simulink model "Total_B2B_latest"  (R2018a)
settings: Solver=ode8  StartTime=0.0  StopTime=10  FixedStep=20e-6  RelTol=1e-3
values from neighbouring files (symbols this model uses):
  A = R^2*pi    (= 24996.5217713)    [Total_init.m]    (also in Total_init_trafo.m)
  C1 = 0.0117    [Total_init.m]    (also in Total_init_trafo.m)
  C2 = 5500    [Total_init.m]    (also in Total_init_trafo.m)
  C3 = 10    [Total_init.m]    (also in Total_init_trafo.m)
  C4 = 0    [Total_init.m]    (also in Total_init_trafo.m)
  C5 = 160    [Total_init.m]    (also in Total_init_trafo.m)
  C6 = 23.38    [Total_init.m]    (also in Total_init_trafo.m)
  C_dc = 1e-2    (= 0.01)    [Total_init.m]    (also in Total_init_trafo.m)
  Cx = 0    [Total_init.m]    (also in Total_init_trafo.m)
  fg = 50    [Total_init.m]    (also in Total_init_trafo.m)
  Ir = 2*Pr/(3*Er*cosphi)    (= 2057.61316872)    [Total_init.m]    (also in Total_init_trafo.m)
  J = 12.8e6    (= 12800000)    [Total_init.m]    (also in Total_init_trafo.m)
  Jr = 3*m*r^2    (= 105248711.1)    [Total_init.m]    (also in Total_init_trafo.m)
  KI_d = KP_d*Rs/Ld    (= 1454)    [Total_init.m]    (also in Total_init_trafo.m)
  KP_d = 50    [Total_init.m]    (also in Total_init_trafo.m)
  KP_g = 5    [Total_init.m]    (also in Total_init_trafo.m)
  KP_gv = 5    [Total_init.m]    (also in Total_init_trafo.m)
  lambda_m = Er/(om_r*p)    (= 21.4859173174)    [Total_init.m]    (also in Total_init_trafo.m)
  lambda_opt = 9.35    [Total_init.m]    (also in Total_init_trafo.m)
  Ld = 0.005    [Total_init.m]    (also in Total_init_trafo.m)
  Lg = 1e-3    (= 0.001)    [Total_init.m]    (also in Total_init_trafo.m)
  Linvmat = Lmat^(-1)    [Total_init.m]    (also in Total_init_trafo.m)
  Lq = 0.005    [Total_init.m]    (also in Total_init_trafo.m)
  om0 = om_r    (= 1.0471975512)    [Total_init.m]    (also in Total_init_trafo.m)
  om_g = 100*pi    (= 314.159265359)    [Total_init.m]    (also in Total_init_trafo.m)
  om_r = 10/60*2*pi    (= 1.0471975512)    [Total_init.m]    (also in Total_init_trafo.m)
  p = 160    [Total_init.m]    (also in Total_init_trafo.m)
  Pr = 10e6    (= 10000000)    [Total_init.m]    (also in Total_init_trafo.m)
  psi0 = Lmat*I0'+psif    [Total_init.m]    (also in Total_init_trafo.m)
  psif = [lambda_m; 0]    [Total_init.m]    (also in Total_init_trafo.m)
  R = 89.2    [Total_init.m]    (also in Total_init_trafo.m)
  R_cs = 1e9    (= 1000000000)    [Total_init.m]    (also in Total_init_trafo.m)
  R_dc = 1e-3    (= 0.001)    [Total_init.m]    (also in Total_init_trafo.m)
  Rg = 1e-6    (= 1e-06)    [Total_init.m]    (also in Total_init_trafo.m)
  rho = 1.225    [Total_init.m]    (also in Total_init_trafo.m)
  Rmat = [Rs 0;         0 Rs]    [Total_init.m]    (also in Total_init_trafo.m)
  Rs = 0.1454    [Total_init.m]    (also in Total_init_trafo.m)
  ts = 0.0001    [Total_init.m]    (also in Total_init_trafo.m)
  Vac = 4000    [Total_init.m]    (also in Total_init_trafo.m)
  Vdc = Vac*sqrt(3)    [Total_init.m]    (also in Total_init_trafo.m)
  Vgsc = Vac    (= 4000)    [Total_init.m]    (also in Total_init_trafo.m)
libraries: powerlib x18, simulink x9
(part 2 of 2)

== system Total_B2B_latest/B2B+grid/MSC/MSC_Controller/Iq_Control ==
  real : Inport
  ref : Inport  Port=2
  Integrator : Integrator  LimitOutput=on  UpperSaturationLimit=Vac  LowerSaturationLimit=-Vac
  K_I : Gain  Gain=10*Rs/Lq
  K_P : Gain  Gain=10
  Saturation : Saturate  UpperLimit=Vac  LowerLimit=-Vac
  Sum : Sum  Inputs=|-+
  Sum1 : Sum  Inputs=|++
  TuneScope_Iq : Scope  NumInputPorts=3
  out : Outport
  wires:
  real/1 -> TuneScope_Iq/1, Sum/1
  K_I/1 -> Integrator/1
  Sum/1 -> K_P/1, K_I/1
  Integrator/1 -> Sum1/1
  Sum1/1 -> Saturation/1
  K_P/1 -> Sum1/2
  Saturation/1 -> TuneScope_Iq/3, out/1
  ref/1 -> TuneScope_Iq/2, Sum/2

== system Total_B2B_latest/B2B+grid/MSC/MSC_Controller/Modulator ==
  v_albe : Inport
  Add : Sum
  Add1 : Sum  Inputs=-+
  Add2 : Sum  Inputs=+-
  Carrier Wave : simulink/Sources/Repeating Sequence  rep_seq_t=[0 0.5/Fs 1/Fs]  rep_seq_y=[-1 1 -1]
  Compare To Zero : simulink/Logic and Bit Operations/Compare To Zero  relop=>=  OutDataTypeStr=boolean
  Constant : Constant  Value=Vdc/2
  Data Type Conversion : DataTypeConversion
  Gain2 : Gain  Gain=0.5
  Gate assignment : Subsystem
  Product : Product
  albe2abc : Subsystem
  max : MinMax  Function=max
  min : MinMax
  Out1 : Outport
  wires:
  Gate assignment/1(G) -> Out1/1
  min/1 -> Add/2
  max/1 -> Add/1
  Add/1 -> Gain2/1
  Gain2/1 -> Add1/1
  Add2/1 -> Compare To Zero/1
  Constant/1 -> Product/2
  Carrier Wave/1 -> Product/1
  albe2abc/1(abc) -> Add1/2, min/1, max/1
  Product/1 -> Add2/2
  v_albe/1 -> albe2abc/1(a+bj)
  Compare To Zero/1 -> Data Type Conversion/1
  Data Type Conversion/1 -> Gate assignment/1(E)
  Add1/1 -> Add2/1

== system Total_B2B_latest/B2B+grid/MSC/MSC_Controller/Speed_Control ==
  ref : Inport
  real : Inport  Port=2
  Integrator : Integrator  LimitOutput=on  UpperSaturationLimit=Ir  LowerSaturationLimit=-Ir
  K_I : Gain  Gain=1e4
  K_P : Gain  Gain=2e4
  Saturation : Saturate  UpperLimit=Ir  LowerLimit=-Ir
  Sum : Sum  Inputs=|-+
  Sum1 : Sum  Inputs=|++
  TuneScope_w : Scope  NumInputPorts=3
  out : Outport
  wires:
  ref/1 -> Sum/2, TuneScope_w/1
  real/1 -> TuneScope_w/2, Sum/1
  K_I/1 -> Integrator/1
  Sum/1 -> K_P/1, K_I/1
  Integrator/1 -> Sum1/1
  Sum1/1 -> Saturation/1
  K_P/1 -> Sum1/2
  Saturation/1 -> TuneScope_w/3, out/1

== system Total_B2B_latest/B2B+grid/GSC/GSC_Modulator1/Modulator/Gate assignment ==
  E : Inport
  Constant : Constant
  Demux : Demux  Outputs=3
  Demux1 : Demux  Outputs=3
  Mux : Mux  Inputs=6
  Sum1 : Sum  Inputs=-+|  SaturateOnIntegerOverflow=on  InputSameDT=on  OutDataTypeStr=Inherit: Same as first input
  G : Outport
  wires:
  Demux/3 -> Mux/5  "C(high)"
  Demux1/3 -> Mux/6  "C(low)"
  Mux/1 -> G/1
  Sum1/1 -> Demux1/1
  E/1 -> Sum1/1, Demux/1
  Constant/1 -> Sum1/2
  Demux/1 -> Mux/1  "A(high)"
  Demux/2 -> Mux/3  "B(high)"
  Demux1/2 -> Mux/4  "B(low)"
  Demux1/1 -> Mux/2  "A(low)"

== system Total_B2B_latest/B2B+grid/GSC/GSC_Modulator1/Modulator/albe2abc ==
  a+bj : Inport
  Gain : Gain  Gain=[1, 0; -0.5, sqrt(3)/2; -0.5, -sqrt(3)/2 ]  Multiplication=Matrix(K*u) (u vector)
  abc : Outport
  wires:
  Gain/1 -> abc/1
  a+bj/1 -> Gain/1

== system Total_B2B_latest/B2B+grid/GSC/GSC_Modulator1/abc->dq/C_rot ==
  in_1 : Inport
  in_3 : Inport  Port=2
  Demux : Demux  Outputs=2
  Product{,1..3} (4 alike) : Product  SaturateOnIntegerOverflow=on  RndMeth=Zero  InputSameDT=on  OutDataTypeStr=Inherit: Same as first input
  Sum : Sum  Inputs=+-  SaturateOnIntegerOverflow=on  InputSameDT=on  OutDataTypeStr=Inherit: Same as first input
  Sum1 : Sum  SaturateOnIntegerOverflow=on  InputSameDT=on  OutDataTypeStr=Inherit: Same as first input
  cos : Fcn  Expr=cos(u(1))
  sin : Fcn  Expr=sin(u(1))
  out_1 : Outport
  out_2 : Outport  Port=2
  wires:
  Demux/2 -> Product/1, Product2/1
  Demux/1 -> Product3/1, Product1/1
  Sum1/1 -> out_2/1
  Sum/1 -> out_1/1
  cos/1 -> Product/2, Product1/2
  sin/1 -> Product3/2, Product2/2
  in_3/1 -> sin/1, cos/1
  Product/1 -> Sum1/2
  Product1/1 -> Sum/1
  Product3/1 -> Sum1/1
  Product2/1 -> Sum/2
  in_1/1 -> Demux/1

== system Total_B2B_latest/B2B+grid/GSC/GSC_Modulator1/abc->dq/abc-ab ==
  abc : Inport
  3 naar 2 : Subsystem
  Demux : Demux  Outputs=3
  Mux : Mux  Inputs=2
  ab : Outport
  wires:
  abc/1 -> Demux/1
  Demux/1 -> 3 naar 2/1(in_1)
  Demux/2 -> 3 naar 2/2(in_2)
  Demux/3 -> 3 naar 2/3(in_3)
  3 naar 2/1(out_1) -> Mux/1
  3 naar 2/2(out_2) -> Mux/2
  Mux/1 -> ab/1

== system Total_B2B_latest/B2B+grid/GSC/GSC_Modulator1/abc->dq1/C_rot ==
  in_1 : Inport
  in_3 : Inport  Port=2
  Demux : Demux  Outputs=2
  Product{,1..3} (4 alike) : Product  SaturateOnIntegerOverflow=on  RndMeth=Zero  InputSameDT=on  OutDataTypeStr=Inherit: Same as first input
  Sum : Sum  Inputs=+-  SaturateOnIntegerOverflow=on  InputSameDT=on  OutDataTypeStr=Inherit: Same as first input
  Sum1 : Sum  SaturateOnIntegerOverflow=on  InputSameDT=on  OutDataTypeStr=Inherit: Same as first input
  cos : Fcn  Expr=cos(u(1))
  sin : Fcn  Expr=sin(u(1))
  out_1 : Outport
  out_2 : Outport  Port=2
  wires:
  Demux/2 -> Product/1, Product2/1
  Demux/1 -> Product3/1, Product1/1
  Sum1/1 -> out_2/1
  Sum/1 -> out_1/1
  cos/1 -> Product/2, Product1/2
  sin/1 -> Product3/2, Product2/2
  in_3/1 -> sin/1, cos/1
  Product/1 -> Sum1/2
  Product1/1 -> Sum/1
  Product3/1 -> Sum1/1
  Product2/1 -> Sum/2
  in_1/1 -> Demux/1

== system Total_B2B_latest/B2B+grid/GSC/GSC_Modulator1/abc->dq1/abc-ab ==
  abc : Inport
  3 naar 2 : Subsystem
  Demux : Demux  Outputs=3
  Mux : Mux  Inputs=2
  ab : Outport
  wires:
  abc/1 -> Demux/1
  Demux/1 -> 3 naar 2/1(in_1)
  Demux/2 -> 3 naar 2/2(in_2)
  Demux/3 -> 3 naar 2/3(in_3)
  3 naar 2/1(out_1) -> Mux/1
  3 naar 2/2(out_2) -> Mux/2
  Mux/1 -> ab/1

== system Total_B2B_latest/B2B+grid/GSC/GSC_Modulator1/dq->ab/C_rot ==
  in_1 : Inport
  in_3 : Inport  Port=2
  Demux : Demux  Outputs=2
  Product{,1..3} (4 alike) : Product  SaturateOnIntegerOverflow=on  RndMeth=Zero  InputSameDT=on  OutDataTypeStr=Inherit: Same as first input
  Sum : Sum  Inputs=+-  SaturateOnIntegerOverflow=on  InputSameDT=on  OutDataTypeStr=Inherit: Same as first input
  Sum1 : Sum  SaturateOnIntegerOverflow=on  InputSameDT=on  OutDataTypeStr=Inherit: Same as first input
  cos : Fcn  Expr=cos(u(1))
  sin : Fcn  Expr=sin(u(1))
  out_1 : Outport
  out_2 : Outport  Port=2
  wires:
  Demux/2 -> Product/1, Product2/1
  Demux/1 -> Product3/1, Product1/1
  Sum1/1 -> out_2/1
  Sum/1 -> out_1/1
  cos/1 -> Product/2, Product1/2
  sin/1 -> Product3/2, Product2/2
  in_3/1 -> sin/1, cos/1
  Product/1 -> Sum1/2
  Product1/1 -> Sum/1
  Product3/1 -> Sum1/1
  Product2/1 -> Sum/2
  in_1/1 -> Demux/1

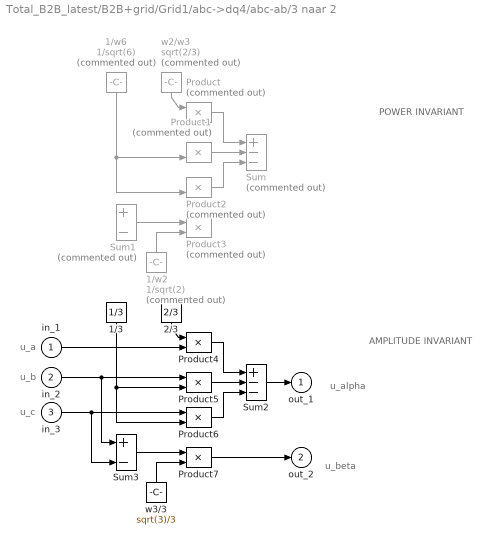
== system Total_B2B_latest/B2B+grid/Grid1/abc->dq4/abc-ab/3 naar 2 ==
  note: POWER INVARIANT
  note: AMPLITUDE INVARIANT
  note: u_beta
  note: u_alpha
  note: u_a
  note: u_c
  note: u_b
  in_1 : Inport
  in_2 : Inport  Port=2
  in_3 : Inport  Port=3
  1/3 : Constant  Value=1/3
  1/w2 : Constant  Commented=on  Value=1/sqrt(2)
  1/w6 : Constant  Commented=on  Value=1/sqrt(6)
  2/3 : Constant  Value=2/3
  Product{,1..3} (4 alike) : Product  Commented=on  SaturateOnIntegerOverflow=on  RndMeth=Zero  InputSameDT=on  OutDataTypeStr=Inherit: Same as first input
  Product{4..7} (4 alike) : Product  SaturateOnIntegerOverflow=on  RndMeth=Zero  InputSameDT=on  OutDataTypeStr=Inherit: Same as first input
  Sum : Sum  Commented=on  Inputs=+--  SaturateOnIntegerOverflow=on  InputSameDT=on  OutDataTypeStr=Inherit: Same as first input
  Sum1 : Sum  Commented=on  Inputs=+-  SaturateOnIntegerOverflow=on  InputSameDT=on  OutDataTypeStr=Inherit: Same as first input
  Sum2 : Sum  Inputs=+--  SaturateOnIntegerOverflow=on  InputSameDT=on  OutDataTypeStr=Inherit: Same as first input
  Sum3 : Sum  Inputs=+-  SaturateOnIntegerOverflow=on  InputSameDT=on  OutDataTypeStr=Inherit: Same as first input
  w2/w3 : Constant  Commented=on  Value=sqrt(2/3)
  w3/3 : Constant  Value=sqrt(3)/3
  out_1 : Outport
  out_2 : Outport  Port=2
  wires:
  1/w2/1 -> Product3/2
  Product2/1 -> Sum/3
  Sum1/1 -> Product3/1
  Product1/1 -> Sum/2
  1/w6/1 -> Product1/2, Product2/2
  w2/w3/1 -> Product/1
  Product/1 -> Sum/1
  in_1/1 -> Product4/2
  Product7/1 -> out_2/1
  Product6/1 -> Sum2/3
  in_3/1 -> Sum3/2, Product6/1
  2/3/1 -> Product4/1
  Product4/1 -> Sum2/1
  Product5/1 -> Sum2/2
  1/3/1 -> Product5/2, Product6/2
  in_2/1 -> Product5/1, Sum3/1
  w3/3/1 -> Product7/2
  Sum3/1 -> Product7/1
  Sum2/1 -> out_1/1

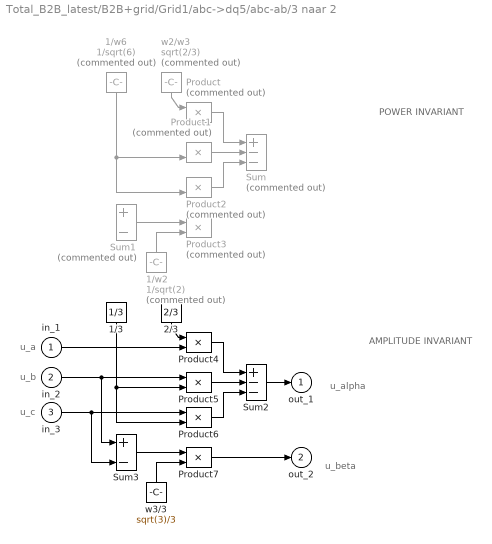
== system Total_B2B_latest/B2B+grid/Grid1/abc->dq5/abc-ab/3 naar 2 ==
  note: POWER INVARIANT
  note: AMPLITUDE INVARIANT
  note: u_beta
  note: u_alpha
  note: u_a
  note: u_c
  note: u_b
  in_1 : Inport
  in_2 : Inport  Port=2
  in_3 : Inport  Port=3
  1/3 : Constant  Value=1/3
  1/w2 : Constant  Commented=on  Value=1/sqrt(2)
  1/w6 : Constant  Commented=on  Value=1/sqrt(6)
  2/3 : Constant  Value=2/3
  Product{,1..3} (4 alike) : Product  Commented=on  SaturateOnIntegerOverflow=on  RndMeth=Zero  InputSameDT=on  OutDataTypeStr=Inherit: Same as first input
  Product{4..7} (4 alike) : Product  SaturateOnIntegerOverflow=on  RndMeth=Zero  InputSameDT=on  OutDataTypeStr=Inherit: Same as first input
  Sum : Sum  Commented=on  Inputs=+--  SaturateOnIntegerOverflow=on  InputSameDT=on  OutDataTypeStr=Inherit: Same as first input
  Sum1 : Sum  Commented=on  Inputs=+-  SaturateOnIntegerOverflow=on  InputSameDT=on  OutDataTypeStr=Inherit: Same as first input
  Sum2 : Sum  Inputs=+--  SaturateOnIntegerOverflow=on  InputSameDT=on  OutDataTypeStr=Inherit: Same as first input
  Sum3 : Sum  Inputs=+-  SaturateOnIntegerOverflow=on  InputSameDT=on  OutDataTypeStr=Inherit: Same as first input
  w2/w3 : Constant  Commented=on  Value=sqrt(2/3)
  w3/3 : Constant  Value=sqrt(3)/3
  out_1 : Outport
  out_2 : Outport  Port=2
  wires:
  1/w2/1 -> Product3/2
  Product2/1 -> Sum/3
  Sum1/1 -> Product3/1
  Product1/1 -> Sum/2
  1/w6/1 -> Product1/2, Product2/2
  w2/w3/1 -> Product/1
  Product/1 -> Sum/1
  in_1/1 -> Product4/2
  Product7/1 -> out_2/1
  Product6/1 -> Sum2/3
  in_3/1 -> Sum3/2, Product6/1
  2/3/1 -> Product4/1
  Product4/1 -> Sum2/1
  Product5/1 -> Sum2/2
  1/3/1 -> Product5/2, Product6/2
  in_2/1 -> Product5/1, Sum3/1
  w3/3/1 -> Product7/2
  Sum3/1 -> Product7/1
  Sum2/1 -> out_1/1

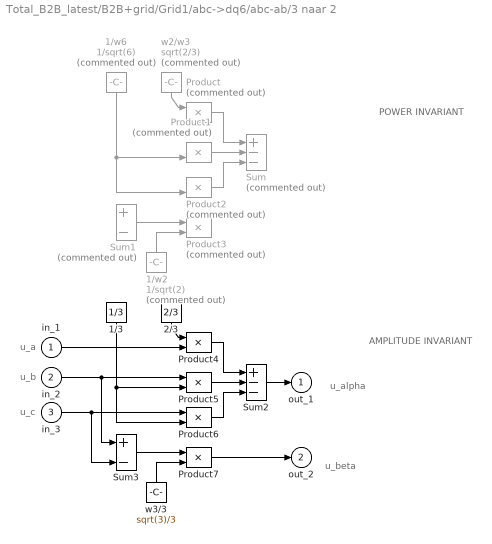
== system Total_B2B_latest/B2B+grid/Grid1/abc->dq6/abc-ab/3 naar 2 ==
  note: POWER INVARIANT
  note: AMPLITUDE INVARIANT
  note: u_beta
  note: u_alpha
  note: u_a
  note: u_c
  note: u_b
  in_1 : Inport
  in_2 : Inport  Port=2
  in_3 : Inport  Port=3
  1/3 : Constant  Value=1/3
  1/w2 : Constant  Commented=on  Value=1/sqrt(2)
  1/w6 : Constant  Commented=on  Value=1/sqrt(6)
  2/3 : Constant  Value=2/3
  Product{,1..3} (4 alike) : Product  Commented=on  SaturateOnIntegerOverflow=on  RndMeth=Zero  InputSameDT=on  OutDataTypeStr=Inherit: Same as first input
  Product{4..7} (4 alike) : Product  SaturateOnIntegerOverflow=on  RndMeth=Zero  InputSameDT=on  OutDataTypeStr=Inherit: Same as first input
  Sum : Sum  Commented=on  Inputs=+--  SaturateOnIntegerOverflow=on  InputSameDT=on  OutDataTypeStr=Inherit: Same as first input
  Sum1 : Sum  Commented=on  Inputs=+-  SaturateOnIntegerOverflow=on  InputSameDT=on  OutDataTypeStr=Inherit: Same as first input
  Sum2 : Sum  Inputs=+--  SaturateOnIntegerOverflow=on  InputSameDT=on  OutDataTypeStr=Inherit: Same as first input
  Sum3 : Sum  Inputs=+-  SaturateOnIntegerOverflow=on  InputSameDT=on  OutDataTypeStr=Inherit: Same as first input
  w2/w3 : Constant  Commented=on  Value=sqrt(2/3)
  w3/3 : Constant  Value=sqrt(3)/3
  out_1 : Outport
  out_2 : Outport  Port=2
  wires:
  1/w2/1 -> Product3/2
  Product2/1 -> Sum/3
  Sum1/1 -> Product3/1
  Product1/1 -> Sum/2
  1/w6/1 -> Product1/2, Product2/2
  w2/w3/1 -> Product/1
  Product/1 -> Sum/1
  in_1/1 -> Product4/2
  Product7/1 -> out_2/1
  Product6/1 -> Sum2/3
  in_3/1 -> Sum3/2, Product6/1
  2/3/1 -> Product4/1
  Product4/1 -> Sum2/1
  Product5/1 -> Sum2/2
  1/3/1 -> Product5/2, Product6/2
  in_2/1 -> Product5/1, Sum3/1
  w3/3/1 -> Product7/2
  Sum3/1 -> Product7/1
  Sum2/1 -> out_1/1

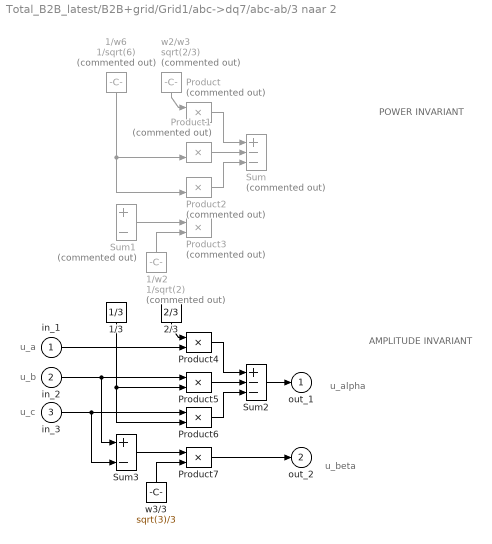
== system Total_B2B_latest/B2B+grid/Grid1/abc->dq7/abc-ab/3 naar 2 ==
  note: POWER INVARIANT
  note: AMPLITUDE INVARIANT
  note: u_beta
  note: u_alpha
  note: u_a
  note: u_c
  note: u_b
  in_1 : Inport
  in_2 : Inport  Port=2
  in_3 : Inport  Port=3
  1/3 : Constant  Value=1/3
  1/w2 : Constant  Commented=on  Value=1/sqrt(2)
  1/w6 : Constant  Commented=on  Value=1/sqrt(6)
  2/3 : Constant  Value=2/3
  Product{,1..3} (4 alike) : Product  Commented=on  SaturateOnIntegerOverflow=on  RndMeth=Zero  InputSameDT=on  OutDataTypeStr=Inherit: Same as first input
  Product{4..7} (4 alike) : Product  SaturateOnIntegerOverflow=on  RndMeth=Zero  InputSameDT=on  OutDataTypeStr=Inherit: Same as first input
  Sum : Sum  Commented=on  Inputs=+--  SaturateOnIntegerOverflow=on  InputSameDT=on  OutDataTypeStr=Inherit: Same as first input
  Sum1 : Sum  Commented=on  Inputs=+-  SaturateOnIntegerOverflow=on  InputSameDT=on  OutDataTypeStr=Inherit: Same as first input
  Sum2 : Sum  Inputs=+--  SaturateOnIntegerOverflow=on  InputSameDT=on  OutDataTypeStr=Inherit: Same as first input
  Sum3 : Sum  Inputs=+-  SaturateOnIntegerOverflow=on  InputSameDT=on  OutDataTypeStr=Inherit: Same as first input
  w2/w3 : Constant  Commented=on  Value=sqrt(2/3)
  w3/3 : Constant  Value=sqrt(3)/3
  out_1 : Outport
  out_2 : Outport  Port=2
  wires:
  1/w2/1 -> Product3/2
  Product2/1 -> Sum/3
  Sum1/1 -> Product3/1
  Product1/1 -> Sum/2
  1/w6/1 -> Product1/2, Product2/2
  w2/w3/1 -> Product/1
  Product/1 -> Sum/1
  in_1/1 -> Product4/2
  Product7/1 -> out_2/1
  Product6/1 -> Sum2/3
  in_3/1 -> Sum3/2, Product6/1
  2/3/1 -> Product4/1
  Product4/1 -> Sum2/1
  Product5/1 -> Sum2/2
  1/3/1 -> Product5/2, Product6/2
  in_2/1 -> Product5/1, Sum3/1
  w3/3/1 -> Product7/2
  Sum3/1 -> Product7/1
  Sum2/1 -> out_1/1

== system Total_B2B_latest/B2B+grid/MSC/MSC_Controller/Modulator/Gate assignment ==
  E : Inport
  Constant : Constant
  Demux : Demux  Outputs=3
  Demux1 : Demux  Outputs=3
  Mux : Mux  Inputs=6
  Sum1 : Sum  Inputs=-+|  SaturateOnIntegerOverflow=on  InputSameDT=on  OutDataTypeStr=Inherit: Same as first input
  G : Outport
  wires:
  Demux/3 -> Mux/5  "C(high)"
  Demux1/3 -> Mux/6  "C(low)"
  Mux/1 -> G/1
  Sum1/1 -> Demux1/1
  E/1 -> Sum1/1, Demux/1
  Constant/1 -> Sum1/2
  Demux/1 -> Mux/1  "A(high)"
  Demux/2 -> Mux/3  "B(high)"
  Demux1/2 -> Mux/4  "B(low)"
  Demux1/1 -> Mux/2  "A(low)"

== system Total_B2B_latest/B2B+grid/MSC/MSC_Controller/Modulator/albe2abc ==
  a+bj : Inport
  Gain : Gain  Gain=[1, 0; -0.5, sqrt(3)/2; -0.5, -sqrt(3)/2 ]  Multiplication=Matrix(K*u) (u vector)
  abc : Outport
  wires:
  Gain/1 -> abc/1
  a+bj/1 -> Gain/1

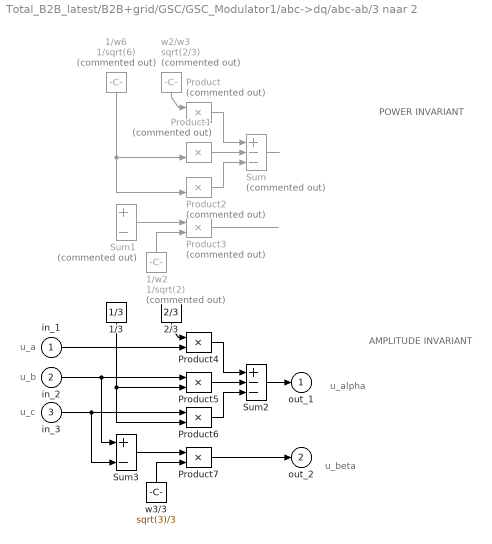
== system Total_B2B_latest/B2B+grid/GSC/GSC_Modulator1/abc->dq/abc-ab/3 naar 2 ==
  note: POWER INVARIANT
  note: AMPLITUDE INVARIANT
  note: u_beta
  note: u_alpha
  note: u_a
  note: u_c
  note: u_b
  in_1 : Inport
  in_2 : Inport  Port=2
  in_3 : Inport  Port=3
  1/3 : Constant  Value=1/3
  1/w2 : Constant  Commented=on  Value=1/sqrt(2)
  1/w6 : Constant  Commented=on  Value=1/sqrt(6)
  2/3 : Constant  Value=2/3
  Product{,1..3} (4 alike) : Product  Commented=on  SaturateOnIntegerOverflow=on  RndMeth=Zero  InputSameDT=on  OutDataTypeStr=Inherit: Same as first input
  Product{4..7} (4 alike) : Product  SaturateOnIntegerOverflow=on  RndMeth=Zero  InputSameDT=on  OutDataTypeStr=Inherit: Same as first input
  Sum : Sum  Commented=on  Inputs=+--  SaturateOnIntegerOverflow=on  InputSameDT=on  OutDataTypeStr=Inherit: Same as first input
  Sum1 : Sum  Commented=on  Inputs=+-  SaturateOnIntegerOverflow=on  InputSameDT=on  OutDataTypeStr=Inherit: Same as first input
  Sum2 : Sum  Inputs=+--  SaturateOnIntegerOverflow=on  InputSameDT=on  OutDataTypeStr=Inherit: Same as first input
  Sum3 : Sum  Inputs=+-  SaturateOnIntegerOverflow=on  InputSameDT=on  OutDataTypeStr=Inherit: Same as first input
  w2/w3 : Constant  Commented=on  Value=sqrt(2/3)
  w3/3 : Constant  Value=sqrt(3)/3
  out_1 : Outport
  out_2 : Outport  Port=2
  wires:
  1/w2/1 -> Product3/2
  Product2/1 -> Sum/3
  Sum1/1 -> Product3/1
  ? -> Sum1/2, Product2/1
  ? -> Product1/1, Sum1/1
  Product1/1 -> Sum/2
  1/w6/1 -> Product1/2, Product2/2
  w2/w3/1 -> Product/1
  Product/1 -> Sum/1
  ? -> Product/2
  Sum/1 -> ?
  Product3/1 -> ?
  in_1/1 -> Product4/2
  Product7/1 -> out_2/1
  Product6/1 -> Sum2/3
  in_3/1 -> Sum3/2, Product6/1
  2/3/1 -> Product4/1
  Product4/1 -> Sum2/1
  Product5/1 -> Sum2/2
  1/3/1 -> Product5/2, Product6/2
  in_2/1 -> Product5/1, Sum3/1
  w3/3/1 -> Product7/2
  Sum3/1 -> Product7/1
  Sum2/1 -> out_1/1

== system Total_B2B_latest/B2B+grid/GSC/GSC_Modulator1/abc->dq1/abc-ab/3 naar 2 ==
  note: POWER INVARIANT
  note: AMPLITUDE INVARIANT
  note: u_beta
  note: u_alpha
  note: u_a
  note: u_c
  note: u_b
  in_1 : Inport
  in_2 : Inport  Port=2
  in_3 : Inport  Port=3
  1/3 : Constant  Value=1/3
  1/w2 : Constant  Value=1/sqrt(2)
  1/w6 : Constant  Value=1/sqrt(6)
  2/3 : Constant  Value=2/3
  Product{,1..7} (8 alike) : Product  SaturateOnIntegerOverflow=on  RndMeth=Zero  InputSameDT=on  OutDataTypeStr=Inherit: Same as first input
  Sum : Sum  Inputs=+--  SaturateOnIntegerOverflow=on  InputSameDT=on  OutDataTypeStr=Inherit: Same as first input
  Sum1 : Sum  Inputs=+-  SaturateOnIntegerOverflow=on  InputSameDT=on  OutDataTypeStr=Inherit: Same as first input
  Sum2 : Sum  Inputs=+--  SaturateOnIntegerOverflow=on  InputSameDT=on  OutDataTypeStr=Inherit: Same as first input
  Sum3 : Sum  Inputs=+-  SaturateOnIntegerOverflow=on  InputSameDT=on  OutDataTypeStr=Inherit: Same as first input
  w2/w3 : Constant  Value=sqrt(2/3)
  w3/3 : Constant  Value=sqrt(3)/3
  out_1 : Outport
  out_2 : Outport  Port=2
  wires:
  1/w2/1 -> Product3/2
  Product2/1 -> Sum/3
  Sum1/1 -> Product3/1
  ? -> Sum1/2, Product2/1
  ? -> Product1/1, Sum1/1
  Product1/1 -> Sum/2
  1/w6/1 -> Product1/2, Product2/2
  w2/w3/1 -> Product/1
  Product/1 -> Sum/1
  ? -> Product/2
  Sum/1 -> ?
  Product3/1 -> ?
  in_1/1 -> Product4/2
  Product7/1 -> out_2/1
  Product6/1 -> Sum2/3
  in_3/1 -> Sum3/2, Product6/1
  2/3/1 -> Product4/1
  Product4/1 -> Sum2/1
  Product5/1 -> Sum2/2
  1/3/1 -> Product5/2, Product6/2
  in_2/1 -> Product5/1, Sum3/1
  w3/3/1 -> Product7/2
  Sum3/1 -> Product7/1
  Sum2/1 -> out_1/1

== matlab function Total_B2B_latest/Rotor/Lambda-Cp1/C_p approx ==
  data: V input; C_p output; pitch input; omega input
function C_p  = fcn(V,pitch,omega)

lambda = omega*89.2/V;

C1 = 0.0117;
C2 = 5500;
C3 = 10;
C4 = 0;
C5 = 160;
C6 = 23.38;
x = 0;

factor = 1/(lambda+0.08*pitch)-0.035/(1+pitch^3);
C_p = C1*(C2*factor-C3/factor*pitch-C4*pitch^x-C5)*exp(-C6*factor);
end
